simulink model "CL_WC"  (R2017a)
settings: Solver=VariableStepAuto  StartTime=0.0  StopTime=450  RelTol=1e-3
values from neighbouring files (symbols this model uses):
  A_new = zeros(6,6)    [main_1.m]
  B_new = zeros(6,2)    [main_1.m]
  C_new = [1 0 0 0 0 0;0 1 0 0 0 0;0 0 1 0 0 0]    [main_1.m]
  D_new = zeros(3,2)    [main_1.m]
libraries: cstblocks x4
settings Model: Creator=Ali  LastModifiedBy=Ali

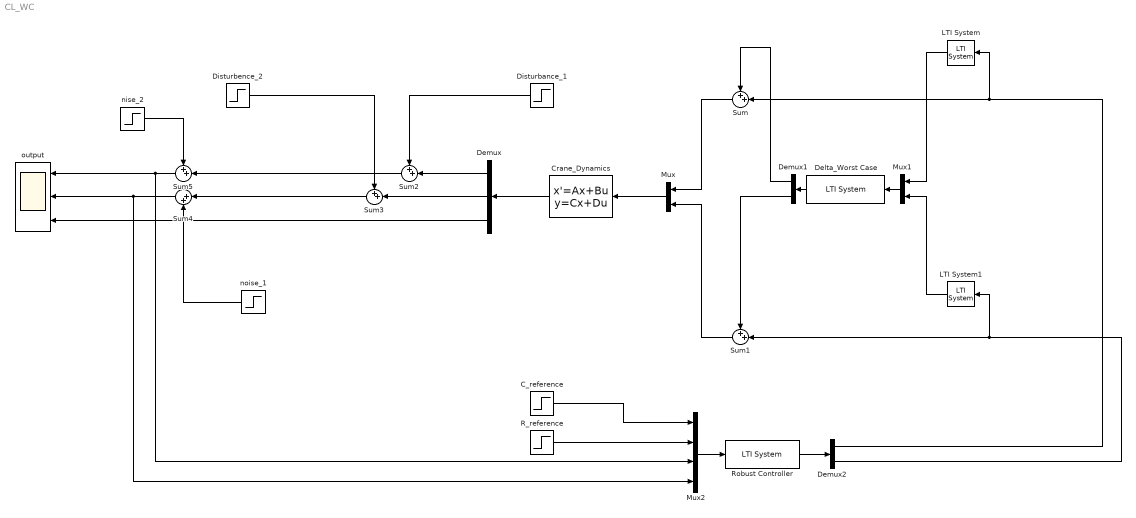
== system CL_WC ==
  C_reference : Step  After=5  SampleTime=0
  Crane_Dynamics : StateSpace  A=A_new  B=B_new  C=C_new  D=D_new  X0=0
  Delta_Worst Case : cstblocks/LTI System  sys=Delta0_wc  IC=[]
  Demux : Demux  Outputs=3
  Demux1 : Demux  Outputs=2
  Demux2 : Demux  Outputs=2
  Disturbance_1 : Step  Time=20  After=5  SampleTime=0
  Disturbence_2 : Step  Time=10  After=-8  SampleTime=0
  LTI System : cstblocks/LTI System  sys=Wa1  IC=[]
  LTI System1 : cstblocks/LTI System  sys=Wa2  IC=[]
  Mux : Mux  Inputs=2
  Mux1 : Mux  Inputs=2
  Mux2 : Mux
  R_reference : Step  After=2  SampleTime=0
  Robust Controller : cstblocks/LTI System  sys=K  IC=[]
  Sum{,1..3,5} (5 alike) : Sum  Inputs=++|
  Sum4 : Sum  Inputs=|++
  nise_2 : Step  Time=35  After=15  SampleTime=0
  noise_1 : Step  Time=5  After=10  SampleTime=0
  output : Scope  NumInputPorts=3
  wires:
  Sum5/1 -> output/1, Mux2/3
  Sum4/1 -> output/2, Mux2/4
  Demux/3 -> output/3
  Sum3/1 -> Sum4/1
  noise_1/1 -> Sum4/2
  Disturbence_2/1 -> Sum3/1
  Demux/2 -> Sum3/2
  Crane_Dynamics/1 -> Demux/1
  Sum2/1 -> Sum5/2
  Demux2/1 -> LTI System/1, Sum/2
  Demux/1 -> Sum2/2
  Sum1/1 -> Mux/2
  Disturbance_1/1 -> Sum2/1
  nise_2/1 -> Sum5/1
  Demux2/2 -> LTI System1/1, Sum1/2
  Sum/1 -> Mux/1
  Mux/1 -> Crane_Dynamics/1
  Mux1/1 -> Delta_Worst Case/1
  Delta_Worst Case/1 -> Demux1/1
  Demux1/1 -> Sum/1
  Demux1/2 -> Sum1/1
  LTI System/1 -> Mux1/1
  LTI System1/1 -> Mux1/2
  Robust Controller/1 -> Demux2/1
  Mux2/1 -> Robust Controller/1
  C_reference/1 -> Mux2/1
  R_reference/1 -> Mux2/2
